simulink model "PTControl"  (Simulink 9.2)
settings: Solver=ode45  StartTime=0.0  StopTime=inf  RelTol=1e-3  EnableMultiTasking=on
libraries: CarMaker4SL x2
(part 2 of 3)

== system PTControl/CarMaker/IPG Vehicle/CarAndTrailer/Forces/Vehicle Forces ==
  Sync_In : Inport
  Bus Creator1 : BusCreator  Inputs=12
  Bus Creator8 : BusCreator  Inputs=16
  BusCreator1 : BusCreator  Inputs=4
  BusCreator2 : BusCreator  Inputs=9
  Demux : Demux  Outputs=16
  Demux1 : Demux  Outputs=12
  Demux2 : Demux  Outputs=13
  Forces : S-Function  FunctionName=CM_Sfun  Parameters='Forces'  SFunctionDeploymentMode=off  EnableBusSupport=off
  Terminator : Terminator
  Sync_Out : Outport
  Car.Virtual : Outport  Port=2
  Car.Aero : Outport  Port=3
  Car.Load : Outport  Port=4
  wires:
  BusCreator1/1 -> Terminator/1  "Aero IF (in)"
  Demux2/13 -> BusCreator2/9  "car Aero Trq_1 z"
  Demux2/12 -> BusCreator2/8  "car Aero Trq_1 y"
  Demux2/11 -> BusCreator2/7  "car Aero Trq_1 x"
  Demux2/10 -> BusCreator2/6  "car Aero Frc_1 z"
  Demux2/9 -> BusCreator2/5  "car Aero Frc_1 y"
  Demux2/8 -> BusCreator2/4  "car Aero Frc_1 x"
  Demux2/7 -> BusCreator2/3  "car Aero PoA_1 z"
  Demux2/6 -> BusCreator2/2  "car Aero PoA_1 y"
  Demux2/5 -> BusCreator2/1  "car Aero PoA_1 x"
  Demux2/4 -> BusCreator1/4  "car Aero tau_1"
  Demux2/3 -> BusCreator1/3  "car Aero ApproachVel_1 z"
  Demux2/2 -> BusCreator1/2  "car Aero ApproachVel_1 y"
  Demux2/1 -> BusCreator1/1  "car Aero ApproachVel_1 x"
  Demux/16 -> Bus Creator8/16  "Car Load_3 tz"
  Demux/15 -> Bus Creator8/15  "Car Load_3 ty"
  Demux/14 -> Bus Creator8/14  "Car Load_3 tx"
  Demux/13 -> Bus Creator8/13  "Car Load_3 mass"
  Demux1/12 -> Bus Creator1/12  "Car Virtual Trq_0 z"
  Demux1/11 -> Bus Creator1/11  "Car Virtual Trq_0 y"
  Demux1/10 -> Bus Creator1/10  "Car Virtual Trq_0 x"
  Demux1/9 -> Bus Creator1/9  "Car Virtual Trq_1 z"
  Demux1/8 -> Bus Creator1/8  "Car Virtual Trq_1 y"
  Demux1/7 -> Bus Creator1/7  "Car Virtual Trq_1 x"
  Demux1/6 -> Bus Creator1/6  "Car Virtual Frc_0 z"
  Demux1/5 -> Bus Creator1/5  "Car Virtual Frc_0 y"
  Demux1/4 -> Bus Creator1/4  "Car Virtual Frc_0 x"
  Sync_In/1 -> Forces/1
  Forces/1 -> Sync_Out/1
  BusCreator2/1 -> Car.Aero/1
  Demux1/1 -> Bus Creator1/1  "Car Virtual Frc_1 x"
  Demux1/2 -> Bus Creator1/2  "Car Virtual Frc_1 y"
  Demux1/3 -> Bus Creator1/3  "Car Virtual Frc_1 z"
  Forces/3 -> Demux2/1
  Forces/2 -> Demux1/1
  Bus Creator1/1 -> Car.Virtual/1
  Bus Creator8/1 -> Car.Load/1
  Demux/1 -> Bus Creator8/1  "Car Load_0 mass"
  Demux/2 -> Bus Creator8/2  "Car Load_0 tx"
  Demux/3 -> Bus Creator8/3  "Car Load_0 ty"
  Demux/4 -> Bus Creator8/4  "Car Load_0 tz"
  Demux/5 -> Bus Creator8/5  "Car Load_1 mass"
  Demux/6 -> Bus Creator8/6  "Car Load_1 tx"
  Demux/7 -> Bus Creator8/7  "Car Load_1 ty"
  Demux/8 -> Bus Creator8/8  "Car Load_1 tz"
  Demux/9 -> Bus Creator8/9  "Car Load_2 mass"
  Demux/10 -> Bus Creator8/10  "Car Load_2 tx"
  Demux/11 -> Bus Creator8/11  "Car Load_2 ty"
  Demux/12 -> Bus Creator8/12  "Car Load_2 tz"
  Forces/4 -> Demux/1

== system PTControl/CarMaker/IPG Vehicle/CarAndTrailer/Trailer/CreateBus Car.Hitch.FrcTrq ==
  In1 : Inport
  Bus Creator7 : BusCreator  Inputs=6
  Demux7 : Demux  Outputs=6
  Out1 : Outport
  wires:
  In1/1 -> Demux7/1
  Bus Creator7/1 -> Out1/1
  Demux7/6 -> Bus Creator7/6  "Car Hitch Trq2Car z"
  Demux7/5 -> Bus Creator7/5  "Car Hitch Trq2Car y"
  Demux7/4 -> Bus Creator7/4  "Car Hitch Trq2Car x"
  Demux7/3 -> Bus Creator7/3  "Car Hitch Frc2Car z"
  Demux7/2 -> Bus Creator7/2  "Car Hitch Frc2Car y"
  Demux7/1 -> Bus Creator7/1  "Car Hitch Frc2Car x"

== system PTControl/CarMaker/IPG Vehicle/CarAndTrailer/Trailer/CreateBus Vhcl.Motion ==
  In1 : Inport
  BusCreator : BusCreator  Inputs=15
  Demux : Demux  Outputs=15
  Out1 : Outport
  wires:
  Demux/15 -> BusCreator/15  "Vhcl YawAcc"
  Demux/14 -> BusCreator/14  "Vhcl YawVel"
  Demux/13 -> BusCreator/13  "Vhcl Yaw"
  Demux/12 -> BusCreator/12  "Vhcl PitchAcc"
  Demux/11 -> BusCreator/11  "Vhcl PitchVel"
  Demux/10 -> BusCreator/10  "Vhcl Pitch"
  Demux/9 -> BusCreator/9  "Vhcl RollAcc"
  Demux/8 -> BusCreator/8  "Vhcl RollVel"
  Demux/7 -> BusCreator/7  "Vhcl Roll"
  Demux/6 -> BusCreator/6  "Vhcl Hitch_Pos z"
  Demux/5 -> BusCreator/5  "Vhcl Hitch_Pos y"
  Demux/4 -> BusCreator/4  "Vhcl Hitch_Pos x"
  Demux/3 -> BusCreator/3  "Vhcl sRoad"
  Demux/2 -> BusCreator/2  "Vhcl Distance"
  Demux/1 -> BusCreator/1  "Vhcl v"
  In1/1 -> Demux/1
  BusCreator/1 -> Out1/1

== system PTControl/CarMaker/IPG Vehicle/CarAndTrailer/Trailer/CreateBus Vhcl.PoI ==
  In1 : Inport
  Bus Creator3 : BusCreator  Inputs=18
  Demux3 : Demux  Outputs=18
  Out1 : Outport
  wires:
  Demux3/18 -> Bus Creator3/18  "Vhcl PoI_GCS Elev"
  Demux3/17 -> Bus Creator3/17  "Vhcl PoI_GCS Lat"
  Demux3/16 -> Bus Creator3/16  "Vhcl PoI_GCS Long"
  Demux3/15 -> Bus Creator3/15  "Vhcl PoI_Acc_1 z"
  Demux3/14 -> Bus Creator3/14  "Vhcl PoI_Acc_1 y"
  Demux3/13 -> Bus Creator3/13  "Vhcl PoI_Acc_1 x"
  Demux3/12 -> Bus Creator3/12  "Vhcl PoI_Vel_1 z"
  Demux3/11 -> Bus Creator3/11  "Vhcl PoI_Vel_1 y"
  Demux3/10 -> Bus Creator3/10  "Vhcl PoI_Vel_1 x"
  Demux3/9 -> Bus Creator3/9  "Vhcl PoI_Acc z"
  Demux3/8 -> Bus Creator3/8  "Vhcl PoI_Acc y"
  Demux3/7 -> Bus Creator3/7  "Vhcl PoI_Acc x"
  Demux3/6 -> Bus Creator3/6  "Vhcl PoI_Vel z"
  Demux3/5 -> Bus Creator3/5  "Vhcl PoI_Vel y"
  Demux3/4 -> Bus Creator3/4  "Vhcl PoI_Vel x"
  Demux3/3 -> Bus Creator3/3  "Vhcl PoI_Pos z"
  Demux3/2 -> Bus Creator3/2  "Vhcl PoI_Pos y"
  In1/1 -> Demux3/1
  Bus Creator3/1 -> Out1/1
  Demux3/1 -> Bus Creator3/1  "Vhcl PoI_Pos x"

== system PTControl/CarMaker/IPG Vehicle/CarAndTrailer/Trailer/CreateBus Vhcl.Steering ==
  In1 : Inport
  Bus Creator3 : BusCreator  Inputs=4
  Demux : Demux
  Out1 : Outport
  wires:
  Bus Creator3/1 -> Out1/1
  Demux/1 -> Bus Creator3/1  "Vhcl Steering Ang"
  Demux/3 -> Bus Creator3/3  "Vhcl Steering AngAcc"
  Demux/2 -> Bus Creator3/2  "Vhcl Steering AngVel"
  Demux/4 -> Bus Creator3/4  "Vhcl Steering Trq"
  In1/1 -> Demux/1

== system PTControl/CarMaker/IPG Vehicle/CarAndTrailer/Trailer/CreateBus Vhcl.Wheel.FL ==
  In1 : Inport
  Bus Creator3 : BusCreator  Inputs=14
  Demux3 : Demux  Outputs=14
  Out1 : Outport
  wires:
  Demux3/14 -> Bus Creator3/14  "Vhcl Wheel FL Trq_WhlBearing"
  Demux3/13 -> Bus Creator3/13  "Vhcl Wheel FL Trq_T2W"
  Demux3/12 -> Bus Creator3/12  "Vhcl Wheel FL SideSlip"
  Demux3/11 -> Bus Creator3/11  "Vhcl Wheel FL LongSlip"
  Demux3/10 -> Bus Creator3/10  "Vhcl Wheel FL vBelt"
  Demux3/9 -> Bus Creator3/9  "Vhcl Wheel FL Fz"
  Demux3/8 -> Bus Creator3/8  "Vhcl Wheel FL Fy"
  Demux3/7 -> Bus Creator3/7  "Vhcl Wheel FL Fx"
  Demux3/6 -> Bus Creator3/6  "Vhcl Wheel FL r_zxy z"
  Demux3/5 -> Bus Creator3/5  "Vhcl Wheel FL r_zxy y"
  Demux3/4 -> Bus Creator3/4  "Vhcl Wheel FL r_zxy x"
  Demux3/3 -> Bus Creator3/3  "Vhcl Wheel FL t z"
  Demux3/2 -> Bus Creator3/2  "Vhcl Wheel FL t y"
  In1/1 -> Demux3/1
  Bus Creator3/1 -> Out1/1
  Demux3/1 -> Bus Creator3/1  "Vhcl Wheel FL t x"

== system PTControl/CarMaker/IPG Vehicle/CarAndTrailer/Trailer/CreateBus Vhcl.Wheel.FR ==
  In1 : Inport
  Bus Creator3 : BusCreator  Inputs=14
  Demux3 : Demux  Outputs=14
  Out1 : Outport
  wires:
  Demux3/14 -> Bus Creator3/14  "Vhcl Wheel FR Trq_WhlBearing"
  Demux3/13 -> Bus Creator3/13  "Vhcl Wheel FR Trq_T2W"
  Demux3/12 -> Bus Creator3/12  "Vhcl Wheel FR SideSlip"
  Demux3/11 -> Bus Creator3/11  "Vhcl Wheel FR LongSlip"
  Demux3/10 -> Bus Creator3/10  "Vhcl Wheel FR vBelt"
  Demux3/9 -> Bus Creator3/9  "Vhcl Wheel FR Fz"
  Demux3/8 -> Bus Creator3/8  "Vhcl Wheel FR Fy"
  Demux3/7 -> Bus Creator3/7  "Vhcl Wheel FR Fx"
  Demux3/6 -> Bus Creator3/6  "Vhcl Wheel FR r_zxy z"
  Demux3/5 -> Bus Creator3/5  "Vhcl Wheel FR r_zxy y"
  Demux3/4 -> Bus Creator3/4  "Vhcl Wheel FR r_zxy x"
  Demux3/3 -> Bus Creator3/3  "Vhcl Wheel FR t z"
  Demux3/2 -> Bus Creator3/2  "Vhcl Wheel FR t y"
  In1/1 -> Demux3/1
  Bus Creator3/1 -> Out1/1
  Demux3/1 -> Bus Creator3/1  "Vhcl Wheel FR t x"

== system PTControl/CarMaker/IPG Vehicle/CarAndTrailer/Trailer/CreateBus Vhcl.Wheel.RL ==
  In1 : Inport
  Bus Creator3 : BusCreator  Inputs=14
  Demux3 : Demux  Outputs=14
  Out1 : Outport
  wires:
  Demux3/14 -> Bus Creator3/14  "Vhcl Wheel RL Trq_WhlBearing"
  Demux3/13 -> Bus Creator3/13  "Vhcl Wheel RL Trq_T2W"
  Demux3/12 -> Bus Creator3/12  "Vhcl Wheel RL SideSlip"
  Demux3/11 -> Bus Creator3/11  "Vhcl Wheel RL LongSlip"
  Demux3/10 -> Bus Creator3/10  "Vhcl Wheel RL vBelt"
  Demux3/9 -> Bus Creator3/9  "Vhcl Wheel RL Fz"
  Demux3/8 -> Bus Creator3/8  "Vhcl Wheel RL Fy"
  Demux3/7 -> Bus Creator3/7  "Vhcl Wheel RL Fx"
  Demux3/6 -> Bus Creator3/6  "Vhcl Wheel RL r_zxy z"
  Demux3/5 -> Bus Creator3/5  "Vhcl Wheel RL r_zxy y"
  Demux3/4 -> Bus Creator3/4  "Vhcl Wheel RL r_zxy x"
  Demux3/3 -> Bus Creator3/3  "Vhcl Wheel RL t z"
  Demux3/2 -> Bus Creator3/2  "Vhcl Wheel RL t y"
  In1/1 -> Demux3/1
  Bus Creator3/1 -> Out1/1
  Demux3/1 -> Bus Creator3/1  "Vhcl Wheel RL t x"

== system PTControl/CarMaker/IPG Vehicle/CarAndTrailer/Trailer/CreateBus Vhcl.Wheel.RR ==
  In1 : Inport
  Bus Creator3 : BusCreator  Inputs=14
  Demux3 : Demux  Outputs=14
  Out1 : Outport
  wires:
  Demux3/14 -> Bus Creator3/14  "Vhcl Wheel RR Trq_WhlBearing"
  Demux3/13 -> Bus Creator3/13  "Vhcl Wheel RR Trq_T2W"
  Demux3/12 -> Bus Creator3/12  "Vhcl Wheel RR SideSlip"
  Demux3/11 -> Bus Creator3/11  "Vhcl Wheel RR LongSlip"
  Demux3/10 -> Bus Creator3/10  "Vhcl Wheel RR vBelt"
  Demux3/9 -> Bus Creator3/9  "Vhcl Wheel RR Fz"
  Demux3/8 -> Bus Creator3/8  "Vhcl Wheel RR Fy"
  Demux3/7 -> Bus Creator3/7  "Vhcl Wheel RR Fx"
  Demux3/6 -> Bus Creator3/6  "Vhcl Wheel RR r_zxy z"
  Demux3/5 -> Bus Creator3/5  "Vhcl Wheel RR r_zxy y"
  Demux3/4 -> Bus Creator3/4  "Vhcl Wheel RR r_zxy x"
  Demux3/3 -> Bus Creator3/3  "Vhcl Wheel RR t z"
  Demux3/2 -> Bus Creator3/2  "Vhcl Wheel RR t y"
  In1/1 -> Demux3/1
  Bus Creator3/1 -> Out1/1
  Demux3/1 -> Bus Creator3/1  "Vhcl Wheel RR t x"

== system PTControl/CarMaker/IPG Vehicle/PowerTrain/PTControl Example/CreateBus PTC ClutchOut ==
  In : Inport
  BusCreator : BusCreator  Inputs=3
  Demux : Demux  Outputs=3
  Out : Outport
  wires:
  Demux/3 -> BusCreator/3  "PTC ClutchOut Trq_out_trg"
  Demux/2 -> BusCreator/2  "PTC ClutchOut rotv_out_trg"
  Demux/1 -> BusCreator/1  "PTC ClutchOut Pos"
  BusCreator/1 -> Out/1
  In/1 -> Demux/1

== system PTControl/CarMaker/IPG Vehicle/PowerTrain/PTControl Example/CreateBus PTC EngineOut ==
  In : Inport
  BusCreator : BusCreator  Inputs=5
  Demux : Demux  Outputs=5
  Out : Outport
  wires:
  Demux/5 -> BusCreator/5  "PTC EngineOut rotv_trg"
  Demux/4 -> BusCreator/4  "PTC EngineOut Trq_trg"
  Demux/3 -> BusCreator/3  "PTC EngineOut Load"
  Demux/2 -> BusCreator/2  "PTC EngineOut FuelCutOff"
  Demux/1 -> BusCreator/1  "PTC EngineOut set_ISC"
  BusCreator/1 -> Out/1
  In/1 -> Demux/1

== system PTControl/CarMaker/IPG Vehicle/PowerTrain/PTControl Example/CreateBus PTC GearBoxM_Out0 ==
  In : Inport
  BusCreator : BusCreator  Inputs=12
  Demux : Demux  Outputs=12
  Out : Outport
  wires:
  Demux/12 -> BusCreator/12  "PTC GearBoxM_Out0 Clutch_dis Trq_out_trg"
  Demux/11 -> BusCreator/11  "PTC GearBoxM_Out0 Clutch_dis rotv_out_trg"
  Demux/10 -> BusCreator/10  "PTC GearBoxM_Out0 Clutch_dis Pos"
  Demux/9 -> BusCreator/9  "PTC GearBoxM_Out0 Clutch Trq_out_trg"
  Demux/8 -> BusCreator/8  "PTC GearBoxM_Out0 Clutch rotv_out_trg"
  Demux/7 -> BusCreator/7  "PTC GearBoxM_Out0 Clutch Pos"
  Demux/6 -> BusCreator/6  "PTC GearBoxM_Out0 Trq_out_trg"
  Demux/5 -> BusCreator/5  "PTC GearBoxM_Out0 rotv_in_trg"
  Demux/4 -> BusCreator/4  "PTC GearBoxM_Out0 i_trg"
  Demux/3 -> BusCreator/3  "PTC GearBoxM_Out0 set_ParkBrake"
  Demux/2 -> BusCreator/2  "PTC GearBoxM_Out0 GearNoTrg_dis"
  Demux/1 -> BusCreator/1  "PTC GearBoxM_Out0 GearNoTrg"
  BusCreator/1 -> Out/1
  In/1 -> Demux/1

== system PTControl/CarMaker/IPG Vehicle/PowerTrain/PTControl Example/CreateBus PTC GearBoxM_Out1 ==
  In : Inport
  BusCreator : BusCreator  Inputs=12
  Demux : Demux  Outputs=12
  Out : Outport
  wires:
  Demux/12 -> BusCreator/12  "PTC GearBoxM_Out1 Clutch_dis Trq_out_trg"
  Demux/11 -> BusCreator/11  "PTC GearBoxM_Out1 Clutch_dis rotv_out_trg"
  Demux/10 -> BusCreator/10  "PTC GearBoxM_Out1 Clutch_dis Pos"
  Demux/9 -> BusCreator/9  "PTC GearBoxM_Out1 Clutch Trq_out_trg"
  Demux/8 -> BusCreator/8  "PTC GearBoxM_Out1 Clutch rotv_out_trg"
  Demux/7 -> BusCreator/7  "PTC GearBoxM_Out1 Clutch Pos"
  Demux/6 -> BusCreator/6  "PTC GearBoxM_Out1 Trq_out_trg"
  Demux/5 -> BusCreator/5  "PTC GearBoxM_Out1 rotv_in_trg"
  Demux/4 -> BusCreator/4  "PTC GearBoxM_Out1 i_trg"
  Demux/3 -> BusCreator/3  "PTC GearBoxM_Out1 set_ParkBrake"
  Demux/2 -> BusCreator/2  "PTC GearBoxM_Out1 GearNoTrg_dis"
  Demux/1 -> BusCreator/1  "PTC GearBoxM_Out1 GearNoTrg"
  BusCreator/1 -> Out/1
  In/1 -> Demux/1

== system PTControl/CarMaker/IPG Vehicle/PowerTrain/PTControl Example/CreateBus PTC GearBoxM_Out2 ==
  In : Inport
  BusCreator : BusCreator  Inputs=12
  Demux : Demux  Outputs=12
  Out : Outport
  wires:
  Demux/12 -> BusCreator/12  "PTC GearBoxM_Out2 Clutch_dis Trq_out_trg"
  Demux/11 -> BusCreator/11  "PTC GearBoxM_Out2 Clutch_dis rotv_out_trg"
  Demux/10 -> BusCreator/10  "PTC GearBoxM_Out2 Clutch_dis Pos"
  Demux/9 -> BusCreator/9  "PTC GearBoxM_Out2 Clutch Trq_out_trg"
  Demux/8 -> BusCreator/8  "PTC GearBoxM_Out2 Clutch rotv_out_trg"
  Demux/7 -> BusCreator/7  "PTC GearBoxM_Out2 Clutch Pos"
  Demux/6 -> BusCreator/6  "PTC GearBoxM_Out2 Trq_out_trg"
  Demux/5 -> BusCreator/5  "PTC GearBoxM_Out2 rotv_in_trg"
  Demux/4 -> BusCreator/4  "PTC GearBoxM_Out2 i_trg"
  Demux/3 -> BusCreator/3  "PTC GearBoxM_Out2 set_ParkBrake"
  Demux/2 -> BusCreator/2  "PTC GearBoxM_Out2 GearNoTrg_dis"
  Demux/1 -> BusCreator/1  "PTC GearBoxM_Out2 GearNoTrg"
  BusCreator/1 -> Out/1
  In/1 -> Demux/1

== system PTControl/CarMaker/IPG Vehicle/PowerTrain/PTControl Example/CreateBus PTC GearBoxM_Out3 ==
  In : Inport
  BusCreator : BusCreator  Inputs=12
  Demux : Demux  Outputs=12
  Out : Outport
  wires:
  Demux/12 -> BusCreator/12  "PTC GearBoxM_Out3 Clutch_dis Trq_out_trg"
  Demux/11 -> BusCreator/11  "PTC GearBoxM_Out3 Clutch_dis rotv_out_trg"
  Demux/10 -> BusCreator/10  "PTC GearBoxM_Out3 Clutch_dis Pos"
  Demux/9 -> BusCreator/9  "PTC GearBoxM_Out3 Clutch Trq_out_trg"
  Demux/8 -> BusCreator/8  "PTC GearBoxM_Out3 Clutch rotv_out_trg"
  Demux/7 -> BusCreator/7  "PTC GearBoxM_Out3 Clutch Pos"
  Demux/6 -> BusCreator/6  "PTC GearBoxM_Out3 Trq_out_trg"
  Demux/5 -> BusCreator/5  "PTC GearBoxM_Out3 rotv_in_trg"
  Demux/4 -> BusCreator/4  "PTC GearBoxM_Out3 i_trg"
  Demux/3 -> BusCreator/3  "PTC GearBoxM_Out3 set_ParkBrake"
  Demux/2 -> BusCreator/2  "PTC GearBoxM_Out3 GearNoTrg_dis"
  Demux/1 -> BusCreator/1  "PTC GearBoxM_Out3 GearNoTrg"
  BusCreator/1 -> Out/1
  In/1 -> Demux/1

== system PTControl/CarMaker/IPG Vehicle/PowerTrain/PTControl Example/CreateBus PTC GearBoxOut ==
  In : Inport
  BusCreator : BusCreator  Inputs=12
  Demux : Demux  Outputs=12
  Out : Outport
  wires:
  Demux/12 -> BusCreator/12  "PTC GearBoxOut Clutch_dis Trq_out_trg"
  Demux/11 -> BusCreator/11  "PTC GearBoxOut Clutch_dis rotv_out_trg"
  Demux/10 -> BusCreator/10  "PTC GearBoxOut Clutch_dis Pos"
  Demux/9 -> BusCreator/9  "PTC GearBoxOut Clutch Trq_out_trg"
  Demux/8 -> BusCreator/8  "PTC GearBoxOut Clutch rotv_out_trg"
  Demux/7 -> BusCreator/7  "PTC GearBoxOut Clutch Pos"
  Demux/6 -> BusCreator/6  "PTC GearBoxOut Trq_out_trg"
  Demux/5 -> BusCreator/5  "PTC GearBoxOut rotv_in_trg"
  Demux/4 -> BusCreator/4  "PTC GearBoxOut i_trg"
  Demux/3 -> BusCreator/3  "PTC GearBoxOut set_ParkBrake"
  Demux/2 -> BusCreator/2  "PTC GearBoxOut GearNoTrg_dis"
  Demux/1 -> BusCreator/1  "PTC GearBoxOut GearNoTrg"
  BusCreator/1 -> Out/1
  In/1 -> Demux/1

== system PTControl/CarMaker/IPG Vehicle/PowerTrain/PTControl Example/CreateBus PTC ISGOut ==
  In : Inport
  BusCreator : BusCreator  Inputs=3
  Demux : Demux  Outputs=3
  Out : Outport
  wires:
  Demux/3 -> BusCreator/3  "PTC ISGOut rotv_trg"
  Demux/2 -> BusCreator/2  "PTC ISGOut Trq_trg"
  Demux/1 -> BusCreator/1  "PTC ISGOut Load"
  BusCreator/1 -> Out/1
  In/1 -> Demux/1

== system PTControl/CarMaker/IPG Vehicle/PowerTrain/PTControl Example/CreateBus PTC MiscOut ==
  In : Inport
  BusCreator : BusCreator  Inputs=4
  Demux : Demux
  Out : Outport
  wires:
  Demux/4 -> BusCreator/4  "PTC_Out Ignition"
  Demux/3 -> BusCreator/3  "PTC_Out StrategyMode"
  Demux/2 -> BusCreator/2  "PTC_Out OperationError"
  Demux/1 -> BusCreator/1  "PTC_Out OperationState"
  BusCreator/1 -> Out/1
  In/1 -> Demux/1

== system PTControl/CarMaker/IPG Vehicle/PowerTrain/PTControl Example/CreateBus PTC MotorOut0 ==
  In : Inport
  BusCreator : BusCreator  Inputs=3
  Demux : Demux  Outputs=3
  Gain : Gain  Gain=3
  Out : Outport
  wires:
  Demux/3 -> BusCreator/3  "PTC MotorOut0 rotv_trg"
  Demux/1 -> BusCreator/1  "PTC MotorOut0 Load"
  BusCreator/1 -> Out/1
  In/1 -> Demux/1
  Demux/2 -> Gain/1  "PTC MotorOut0 Trq_trg"
  Gain/1 -> BusCreator/2

== system PTControl/CarMaker/IPG Vehicle/PowerTrain/PTControl Example/CreateBus PTC MotorOut1 ==
  In : Inport
  BusCreator : BusCreator  Inputs=3
  Demux : Demux  Outputs=3
  Out : Outport
  wires:
  Demux/3 -> BusCreator/3  "PTC MotorOut1 rotv_trg"
  Demux/2 -> BusCreator/2  "PTC MotorOut1 Trq_trg"
  Demux/1 -> BusCreator/1  "PTC MotorOut1 Load"
  BusCreator/1 -> Out/1
  In/1 -> Demux/1

== system PTControl/CarMaker/IPG Vehicle/PowerTrain/PTControl Example/CreateBus PTC MotorOut2 ==
  In : Inport
  BusCreator : BusCreator  Inputs=3
  Demux : Demux  Outputs=3
  Out : Outport
  wires:
  Demux/3 -> BusCreator/3  "PTC MotorOut2 rotv_trg"
  Demux/2 -> BusCreator/2  "PTC MotorOut2 Trq_trg"
  Demux/1 -> BusCreator/1  "PTC MotorOut2 Load"
  BusCreator/1 -> Out/1
  In/1 -> Demux/1

== system PTControl/CarMaker/IPG Vehicle/PowerTrain/PTControl Example/CreateBus PTC MotorOut3 ==
  In : Inport
  BusCreator : BusCreator  Inputs=3
  Demux : Demux  Outputs=3
  Out : Outport
  wires:
  Demux/3 -> BusCreator/3  "PTC MotorOut3 rotv_trg"
  Demux/2 -> BusCreator/2  "PTC MotorOut3 Trq_trg"
  Demux/1 -> BusCreator/1  "PTC MotorOut3 Load"
  BusCreator/1 -> Out/1
  In/1 -> Demux/1

== system PTControl/CarMaker/IPG Vehicle/PowerTrain/PTControl Example/CreateBus PTC PwrSupplyOut ==
  In : Inport
  BusCreator : BusCreator  Inputs=1
  Demux : Demux  Outputs=1
  Out : Outport
  wires:
  Demux/1 -> BusCreator/1  "PTC PwrSupplyOut Pwr_HV1toLV_trg"
  BusCreator/1 -> Out/1
  In/1 -> Demux/1

== system PTControl/CarMaker/IPG Vehicle/PowerTrain/PTControl Example/CreateBus PTC WheelOut ==
  In : Inport
  BusCreator : BusCreator  Inputs=8
  Demux : Demux  Outputs=8
  Out : Outport
  wires:
  Demux/8 -> BusCreator/8  "PTC WheelOut_RR Trq_BrakeReg_max"
  Demux/7 -> BusCreator/7  "PTC WheelOut_RR Trq_BrakeReg"
  Demux/6 -> BusCreator/6  "PTC WheelOut_RL Trq_BrakeReg_max"
  Demux/5 -> BusCreator/5  "PTC WheelOut_RL Trq_BrakeReg"
  Demux/4 -> BusCreator/4  "PTC WheelOut_FR Trq_BrakeReg_max"
  Demux/3 -> BusCreator/3  "PTC WheelOut_FR Trq_BrakeReg"
  Demux/2 -> BusCreator/2  "PTC WheelOut_FL Trq_BrakeReg_max"
  Demux/1 -> BusCreator/1  "PTC WheelOut_FL Trq_BrakeReg"
  BusCreator/1 -> Out/1
  In/1 -> Demux/1

== system PTControl/CarMaker/IPG Vehicle/PowerTrain/PTControl Example/PTControl Example ==
  note: Minimalistic PTControl example model, that only works with
      | the 'Generic' powertrain and the 'Manual' gearbox.
  EngineIn : Inport
  VhclCtrl.PT : Inport  Port=2
  Bus Selector : BusSelector  OutputSignals=VhclCtrl Key,VhclCtrl Gas,VhclCtrl Clutch,VhclCtrl GearNo
  Bus Selector1 : BusSelector  OutputSignals=PTC EngineIn.PTC EngineIn Engine_on
  Define CM Dict : CarMaker4SL/Define CM Dict  xname=test  xmono=off  xtype=Double4  xdvaplace=None  xnstates=0  xfirststate=0  xinitial=0
  Engine : Subsystem
  ISG : Subsystem
  PTC : Subsystem
  Write CM Dict : CarMaker4SL/Write CM Dict  xname=test  xsync=off
  PTC MiscOut : Outport
  EngineOut : Outport  Port=2
  ISGOut : Outport  Port=3
  ClutchOut Pos : Outport  Port=4
  GearBoxOut GearNoTrg : Outport  Port=5
  wires:
  VhclCtrl.PT/1 -> Bus Selector/1
  EngineIn/1 -> Bus Selector1/1
  Engine/1(EngineOut) -> EngineOut/1
  Bus Selector1/1 -> Engine/2(Engine_on), PTC/2(Engine_on), Write CM Dict/1  "<PTC EngineIn Engine_on>"
  Bus Selector/2 -> Engine/1(Gas)  "<VhclCtrl Gas>"
  ISG/1(ISGOut) -> ISGOut/1
  PTC/1(PTC MiscOut) -> PTC MiscOut/1
  Bus Selector/4 -> GearBoxOut GearNoTrg/1  "<VhclCtrl GearNo>"
  Bus Selector/3 -> ClutchOut Pos/1  "<VhclCtrl Clutch>"
  Bus Selector/1 -> PTC/1(Key), ISG/1(Key)  "<VhclCtrl Key>"

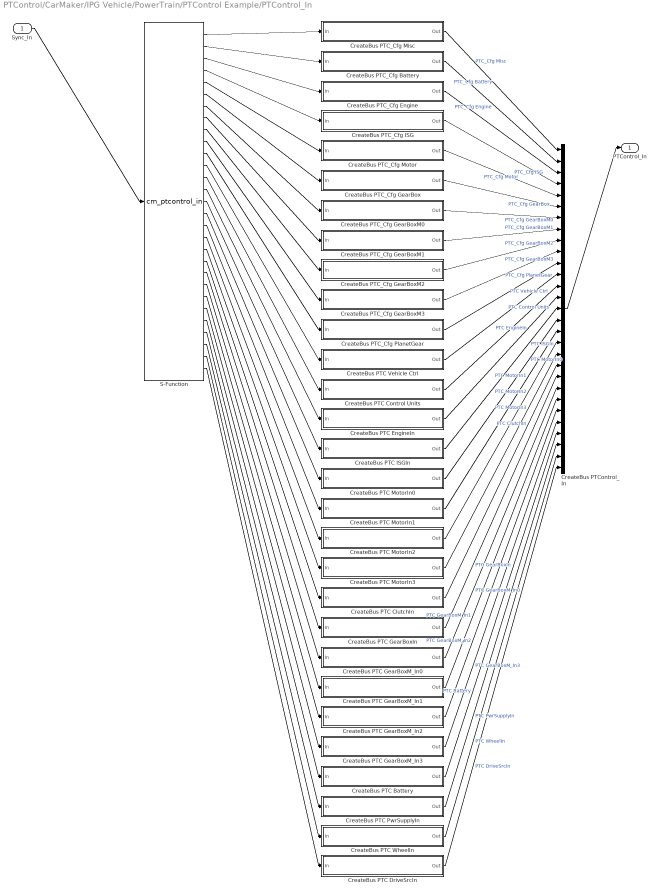
== system PTControl/CarMaker/IPG Vehicle/PowerTrain/PTControl Example/PTControl_In ==
  Sync_In : Inport
  CreateBus PTC Battery : Subsystem
  CreateBus PTC ClutchIn : Subsystem
  CreateBus PTC Control Units : Subsystem
  CreateBus PTC DriveSrcIn : Subsystem
  CreateBus PTC EngineIn : Subsystem
  CreateBus PTC GearBoxIn : Subsystem
  CreateBus PTC GearBoxM_In0 : Subsystem
  CreateBus PTC GearBoxM_In1 : Subsystem
  CreateBus PTC GearBoxM_In2 : Subsystem
  CreateBus PTC GearBoxM_In3 : Subsystem
  CreateBus PTC ISGIn : Subsystem
  CreateBus PTC MotorIn0 : Subsystem
  CreateBus PTC MotorIn1 : Subsystem
  CreateBus PTC MotorIn2 : Subsystem
  CreateBus PTC MotorIn3 : Subsystem
  CreateBus PTC PwrSupplyIn : Subsystem
  CreateBus PTC Vehicle Ctrl : Subsystem
  CreateBus PTC WheelIn : Subsystem
  CreateBus PTC_Cfg Battery : Subsystem
  CreateBus PTC_Cfg Engine : Subsystem
  CreateBus PTC_Cfg GearBox : Subsystem
  CreateBus PTC_Cfg GearBoxM0 : Subsystem
  CreateBus PTC_Cfg GearBoxM1 : Subsystem
  CreateBus PTC_Cfg GearBoxM2 : Subsystem
  CreateBus PTC_Cfg GearBoxM3 : Subsystem
  CreateBus PTC_Cfg ISG : Subsystem
  CreateBus PTC_Cfg Misc : Subsystem
  CreateBus PTC_Cfg Motor : Subsystem
  CreateBus PTC_Cfg PlanetGear : Subsystem
  CreateBus PTControl_In : BusCreator  Inputs=29
  S-Function : S-Function  FunctionName=cm_ptcontrol_in  SFunctionDeploymentMode=off  EnableBusSupport=off
  PTControl_In : Outport
  wires:
  CreateBus PTC DriveSrcIn/1(Out) -> CreateBus PTControl_In/29  "PTC DriveSrcIn"
  S-Function/29 -> CreateBus PTC DriveSrcIn/1(In)
  CreateBus PTC WheelIn/1(Out) -> CreateBus PTControl_In/28  "PTC WheelIn"
  S-Function/28 -> CreateBus PTC WheelIn/1(In)
  CreateBus PTC PwrSupplyIn/1(Out) -> CreateBus PTControl_In/27  "PTC PwrSupplyIn"
  S-Function/27 -> CreateBus PTC PwrSupplyIn/1(In)
  CreateBus PTC Battery/1(Out) -> CreateBus PTControl_In/26  "PTC Battery"
  S-Function/26 -> CreateBus PTC Battery/1(In)
  CreateBus PTC GearBoxM_In3/1(Out) -> CreateBus PTControl_In/25  "PTC GearBoxM_In3"
  S-Function/25 -> CreateBus PTC GearBoxM_In3/1(In)
  CreateBus PTC GearBoxM_In2/1(Out) -> CreateBus PTControl_In/24  "PTC GearBoxM_In2"
  S-Function/24 -> CreateBus PTC GearBoxM_In2/1(In)
  CreateBus PTC GearBoxM_In1/1(Out) -> CreateBus PTControl_In/23  "PTC GearBoxM_In1"
  S-Function/23 -> CreateBus PTC GearBoxM_In1/1(In)
  CreateBus PTC GearBoxM_In0/1(Out) -> CreateBus PTControl_In/22  "PTC GearBoxM_In0"
  S-Function/22 -> CreateBus PTC GearBoxM_In0/1(In)
  CreateBus PTC GearBoxIn/1(Out) -> CreateBus PTControl_In/21  "PTC GearBoxIn"
  S-Function/21 -> CreateBus PTC GearBoxIn/1(In)
  CreateBus PTC ClutchIn/1(Out) -> CreateBus PTControl_In/20  "PTC ClutchIn"
  S-Function/20 -> CreateBus PTC ClutchIn/1(In)
  CreateBus PTC MotorIn3/1(Out) -> CreateBus PTControl_In/19  "PTC MotorIn3"
  S-Function/19 -> CreateBus PTC MotorIn3/1(In)
  CreateBus PTC MotorIn2/1(Out) -> CreateBus PTControl_In/18  "PTC MotorIn2"
  S-Function/18 -> CreateBus PTC MotorIn2/1(In)
  CreateBus PTC MotorIn1/1(Out) -> CreateBus PTControl_In/17  "PTC MotorIn1"
  S-Function/17 -> CreateBus PTC MotorIn1/1(In)
  CreateBus PTC MotorIn0/1(Out) -> CreateBus PTControl_In/16  "PTC MotorIn0"
  S-Function/16 -> CreateBus PTC MotorIn0/1(In)
  CreateBus PTC ISGIn/1(Out) -> CreateBus PTControl_In/15  "PTC ISGIn"
  S-Function/15 -> CreateBus PTC ISGIn/1(In)
  CreateBus PTC EngineIn/1(Out) -> CreateBus PTControl_In/14  "PTC EngineIn"
  S-Function/14 -> CreateBus PTC EngineIn/1(In)
  CreateBus PTC Control Units/1(Out) -> CreateBus PTControl_In/13  "PTC Control Units"
  S-Function/13 -> CreateBus PTC Control Units/1(In)
  CreateBus PTC Vehicle Ctrl/1(Out) -> CreateBus PTControl_In/12  "PTC Vehicle Ctrl"
  S-Function/12 -> CreateBus PTC Vehicle Ctrl/1(In)
  CreateBus PTC_Cfg PlanetGear/1(Out) -> CreateBus PTControl_In/11  "PTC_Cfg PlanetGear"
  S-Function/11 -> CreateBus PTC_Cfg PlanetGear/1(In)
  CreateBus PTC_Cfg GearBoxM3/1(Out) -> CreateBus PTControl_In/10  "PTC_Cfg GearBoxM3"
  S-Function/10 -> CreateBus PTC_Cfg GearBoxM3/1(In)
  CreateBus PTC_Cfg GearBoxM2/1(Out) -> CreateBus PTControl_In/9  "PTC_Cfg GearBoxM2"
  S-Function/9 -> CreateBus PTC_Cfg GearBoxM2/1(In)
  CreateBus PTC_Cfg GearBoxM1/1(Out) -> CreateBus PTControl_In/8  "PTC_Cfg GearBoxM1"
  S-Function/8 -> CreateBus PTC_Cfg GearBoxM1/1(In)
  CreateBus PTC_Cfg GearBoxM0/1(Out) -> CreateBus PTControl_In/7  "PTC_Cfg GearBoxM0"
  S-Function/7 -> CreateBus PTC_Cfg GearBoxM0/1(In)
  CreateBus PTC_Cfg GearBox/1(Out) -> CreateBus PTControl_In/6  "PTC_Cfg GearBox"
  S-Function/6 -> CreateBus PTC_Cfg GearBox/1(In)
  CreateBus PTC_Cfg Motor/1(Out) -> CreateBus PTControl_In/5  "PTC_Cfg Motor"
  S-Function/5 -> CreateBus PTC_Cfg Motor/1(In)
  CreateBus PTC_Cfg ISG/1(Out) -> CreateBus PTControl_In/4  "PTC_Cfg ISG"
  S-Function/4 -> CreateBus PTC_Cfg ISG/1(In)
  CreateBus PTC_Cfg Engine/1(Out) -> CreateBus PTControl_In/3  "PTC_Cfg Engine"
  S-Function/3 -> CreateBus PTC_Cfg Engine/1(In)
  CreateBus PTC_Cfg Battery/1(Out) -> CreateBus PTControl_In/2  "PTC_Cfg Battery"
  S-Function/2 -> CreateBus PTC_Cfg Battery/1(In)
  CreateBus PTC_Cfg Misc/1(Out) -> CreateBus PTControl_In/1  "PTC_Cfg Misc"
  S-Function/1 -> CreateBus PTC_Cfg Misc/1(In)
  CreateBus PTControl_In/1 -> PTControl_In/1
  Sync_In/1 -> S-Function/1

== system PTControl/CarMaker/IPG Vehicle/PowerTrain/PTControl Example/PTControl_Out ==
  PTC MiscOut : Inport
  PTC EngineOut : Inport  Port=2
  PTC ISGOut : Inport  Port=3
  PTC MotorOut0 : Inport  Port=4
  PTC MotorOut1 : Inport  Port=5
  PTC MotorOut2 : Inport  Port=6
  PTC MotorOut3 : Inport  Port=7
  PTC ClutchOut : Inport  Port=8
  PTC GearBoxOut : Inport  Port=9
  PTC GearBoxM_Out0 : Inport  Port=10
  PTC GearBoxM_Out1 : Inport  Port=11
  PTC GearBoxM_Out2 : Inport  Port=12
  PTC GearBoxM_Out3 : Inport  Port=13
  PTC PwrSupplyOut : Inport  Port=14
  PTC WheelOut : Inport  Port=15
  PTControl_Out : S-Function  FunctionName=cm_ptcontrol_out  SFunctionDeploymentMode=off  EnableBusSupport=off
  wires:
  PTC WheelOut/1 -> PTControl_Out/15
  PTC PwrSupplyOut/1 -> PTControl_Out/14
  PTC GearBoxM_Out3/1 -> PTControl_Out/13
  PTC GearBoxM_Out2/1 -> PTControl_Out/12
  PTC GearBoxM_Out1/1 -> PTControl_Out/11
  PTC GearBoxM_Out0/1 -> PTControl_Out/10
  PTC GearBoxOut/1 -> PTControl_Out/9
  PTC ClutchOut/1 -> PTControl_Out/8
  PTC MotorOut3/1 -> PTControl_Out/7
  PTC MotorOut2/1 -> PTControl_Out/6
  PTC MotorOut1/1 -> PTControl_Out/5
  PTC MotorOut0/1 -> PTControl_Out/4
  PTC ISGOut/1 -> PTControl_Out/3
  PTC EngineOut/1 -> PTControl_Out/2
  PTC MiscOut/1 -> PTControl_Out/1

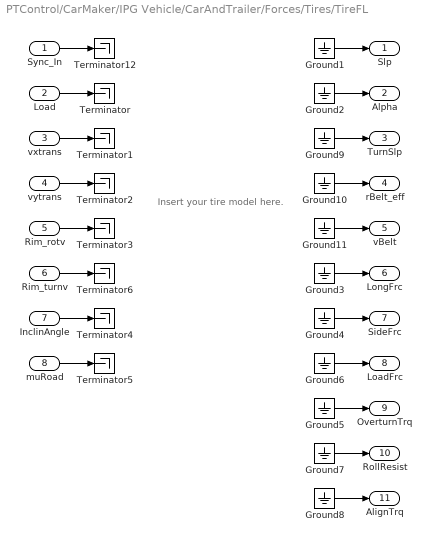
== system PTControl/CarMaker/IPG Vehicle/CarAndTrailer/Forces/Tires/TireFL ==
  note: Insert your tire model here.
  Sync_In : Inport
  Load : Inport  Port=2
  vxtrans : Inport  Port=3
  vytrans : Inport  Port=4
  Rim_rotv : Inport  Port=5
  Rim_turnv : Inport  Port=6
  InclinAngle : Inport  Port=7
  muRoad : Inport  Port=8
  Ground{1..11} (11 alike) : Ground
  Terminator{,1..6,12} (8 alike) : Terminator
  Slp : Outport
  Alpha : Outport  Port=2
  TurnSlp : Outport  Port=3
  rBelt_eff : Outport  Port=4
  vBelt : Outport  Port=5
  LongFrc : Outport  Port=6
  SideFrc : Outport  Port=7
  LoadFrc : Outport  Port=8
  OverturnTrq : Outport  Port=9
  RollResist : Outport  Port=10
  AlignTrq : Outport  Port=11
  wires:
  Ground11/1 -> vBelt/1
  Ground10/1 -> rBelt_eff/1
  Ground9/1 -> TurnSlp/1
  Rim_turnv/1 -> Terminator6/1
  Sync_In/1 -> Terminator12/1
  Ground2/1 -> Alpha/1
  Ground3/1 -> LongFrc/1
  Ground4/1 -> SideFrc/1
  Ground5/1 -> OverturnTrq/1
  vxtrans/1 -> Terminator1/1
  vytrans/1 -> Terminator2/1
  Rim_rotv/1 -> Terminator3/1
  InclinAngle/1 -> Terminator4/1
  muRoad/1 -> Terminator5/1
  Load/1 -> Terminator/1
  Ground1/1 -> Slp/1
  Ground6/1 -> LoadFrc/1
  Ground7/1 -> RollResist/1
  Ground8/1 -> AlignTrq/1

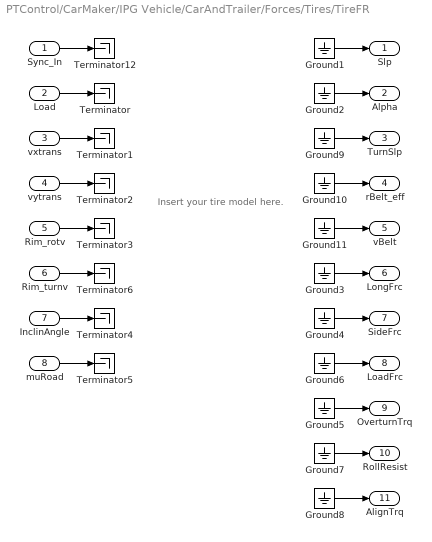
== system PTControl/CarMaker/IPG Vehicle/CarAndTrailer/Forces/Tires/TireFR ==
  note: Insert your tire model here.
  Sync_In : Inport
  Load : Inport  Port=2
  vxtrans : Inport  Port=3
  vytrans : Inport  Port=4
  Rim_rotv : Inport  Port=5
  Rim_turnv : Inport  Port=6
  InclinAngle : Inport  Port=7
  muRoad : Inport  Port=8
  Ground{1..11} (11 alike) : Ground
  Terminator{,1..6,12} (8 alike) : Terminator
  Slp : Outport
  Alpha : Outport  Port=2
  TurnSlp : Outport  Port=3
  rBelt_eff : Outport  Port=4
  vBelt : Outport  Port=5
  LongFrc : Outport  Port=6
  SideFrc : Outport  Port=7
  LoadFrc : Outport  Port=8
  OverturnTrq : Outport  Port=9
  RollResist : Outport  Port=10
  AlignTrq : Outport  Port=11
  wires:
  Ground11/1 -> vBelt/1
  Ground10/1 -> rBelt_eff/1
  Ground9/1 -> TurnSlp/1
  Rim_turnv/1 -> Terminator6/1
  Sync_In/1 -> Terminator12/1
  Ground2/1 -> Alpha/1
  Ground3/1 -> LongFrc/1
  Ground4/1 -> SideFrc/1
  Ground5/1 -> OverturnTrq/1
  vxtrans/1 -> Terminator1/1
  vytrans/1 -> Terminator2/1
  Rim_rotv/1 -> Terminator3/1
  InclinAngle/1 -> Terminator4/1
  muRoad/1 -> Terminator5/1
  Load/1 -> Terminator/1
  Ground1/1 -> Slp/1
  Ground6/1 -> LoadFrc/1
  Ground7/1 -> RollResist/1
  Ground8/1 -> AlignTrq/1

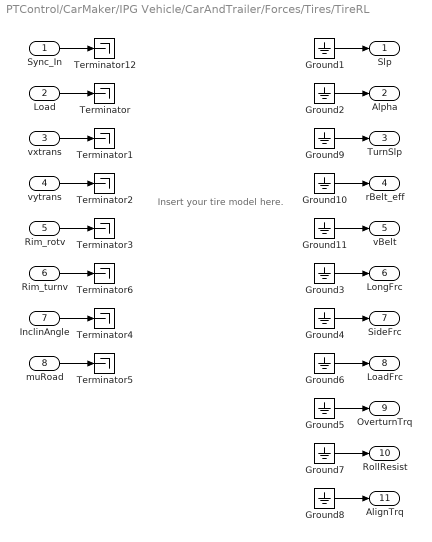
== system PTControl/CarMaker/IPG Vehicle/CarAndTrailer/Forces/Tires/TireRL ==
  note: Insert your tire model here.
  Sync_In : Inport
  Load : Inport  Port=2
  vxtrans : Inport  Port=3
  vytrans : Inport  Port=4
  Rim_rotv : Inport  Port=5
  Rim_turnv : Inport  Port=6
  InclinAngle : Inport  Port=7
  muRoad : Inport  Port=8
  Ground{1..11} (11 alike) : Ground
  Terminator{,1..6,12} (8 alike) : Terminator
  Slp : Outport
  Alpha : Outport  Port=2
  TurnSlp : Outport  Port=3
  rBelt_eff : Outport  Port=4
  vBelt : Outport  Port=5
  LongFrc : Outport  Port=6
  SideFrc : Outport  Port=7
  LoadFrc : Outport  Port=8
  OverturnTrq : Outport  Port=9
  RollResist : Outport  Port=10
  AlignTrq : Outport  Port=11
  wires:
  Ground11/1 -> vBelt/1
  Ground10/1 -> rBelt_eff/1
  Ground9/1 -> TurnSlp/1
  Rim_turnv/1 -> Terminator6/1
  Sync_In/1 -> Terminator12/1
  Ground2/1 -> Alpha/1
  Ground3/1 -> LongFrc/1
  Ground4/1 -> SideFrc/1
  Ground5/1 -> OverturnTrq/1
  vxtrans/1 -> Terminator1/1
  vytrans/1 -> Terminator2/1
  Rim_rotv/1 -> Terminator3/1
  InclinAngle/1 -> Terminator4/1
  muRoad/1 -> Terminator5/1
  Load/1 -> Terminator/1
  Ground1/1 -> Slp/1
  Ground6/1 -> LoadFrc/1
  Ground7/1 -> RollResist/1
  Ground8/1 -> AlignTrq/1

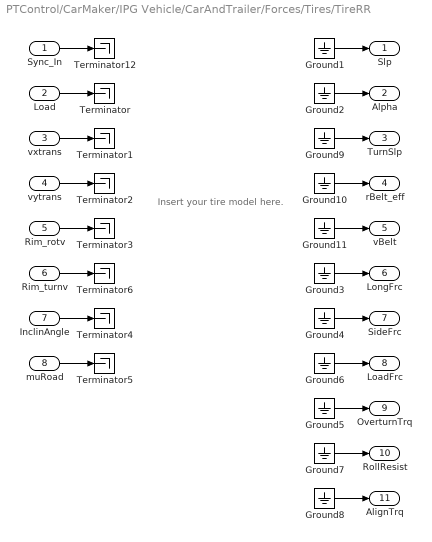
== system PTControl/CarMaker/IPG Vehicle/CarAndTrailer/Forces/Tires/TireRR ==
  note: Insert your tire model here.
  Sync_In : Inport
  Load : Inport  Port=2
  vxtrans : Inport  Port=3
  vytrans : Inport  Port=4
  Rim_rotv : Inport  Port=5
  Rim_turnv : Inport  Port=6
  InclinAngle : Inport  Port=7
  muRoad : Inport  Port=8
  Ground{1..11} (11 alike) : Ground
  Terminator{,1..6,12} (8 alike) : Terminator
  Slp : Outport
  Alpha : Outport  Port=2
  TurnSlp : Outport  Port=3
  rBelt_eff : Outport  Port=4
  vBelt : Outport  Port=5
  LongFrc : Outport  Port=6
  SideFrc : Outport  Port=7
  LoadFrc : Outport  Port=8
  OverturnTrq : Outport  Port=9
  RollResist : Outport  Port=10
  AlignTrq : Outport  Port=11
  wires:
  Ground11/1 -> vBelt/1
  Ground10/1 -> rBelt_eff/1
  Ground9/1 -> TurnSlp/1
  Rim_turnv/1 -> Terminator6/1
  Sync_In/1 -> Terminator12/1
  Ground2/1 -> Alpha/1
  Ground3/1 -> LongFrc/1
  Ground4/1 -> SideFrc/1
  Ground5/1 -> OverturnTrq/1
  vxtrans/1 -> Terminator1/1
  vytrans/1 -> Terminator2/1
  Rim_rotv/1 -> Terminator3/1
  InclinAngle/1 -> Terminator4/1
  muRoad/1 -> Terminator5/1
  Load/1 -> Terminator/1
  Ground1/1 -> Slp/1
  Ground6/1 -> LoadFrc/1
  Ground7/1 -> RollResist/1
  Ground8/1 -> AlignTrq/1

== system PTControl/CarMaker/IPG Vehicle/PowerTrain/PTControl Example/PTControl Example/Engine ==
  Gas : Inport
  Engine_on : Inport  Port=2
  Constant : Constant
  Constant1 : Constant  Value=0
  Constant3 : Constant  Value=0
  Mux : Mux  Inputs=5
  NOTSET0 : Constant  Value=-99999
  NOTSET1 : Constant  Value=-99999
  NOTSET2 : Constant  Value=-99999
  Switch : Switch  Criteria=u2 ~= 0
  Switch1 : Switch  Criteria=u2 ~= 0
  EngineOut : Outport
  wires:
  Constant/1 -> Switch/1
  Mux/1 -> EngineOut/1
  Constant1/1 -> Switch/3
  Engine_on/1 -> Switch/2, Switch1/2
  Gas/1 -> Switch1/1
  Constant3/1 -> Switch1/3
  NOTSET1/1 -> Mux/5  "rotv_trg"
  NOTSET2/1 -> Mux/4  "Trq_trg"
  Switch1/1 -> Mux/3  "Load"
  NOTSET0/1 -> Mux/2  "FuelCutOff"
  Switch/1 -> Mux/1  "set_ISC"

== system PTControl/CarMaker/IPG Vehicle/PowerTrain/PTControl Example/PTControl Example/ISG ==
  Key : Inport
  Constant : Constant
  Constant1 : Constant  Value=0
  KeyPos_KeyIn_Starter : Constant  Value=4
  Mux : Mux  Inputs=3
  NOTSET : Constant  Value=-99999
  NOTSET1 : Constant  Value=-99999
  Relational Operator1 : RelationalOperator  Operator===  OutDataTypeStr=boolean  RndMeth=Nearest
  Switch : Switch  Criteria=u2 ~= 0
  ISGOut : Outport
  wires:
  KeyPos_KeyIn_Starter/1 -> Relational Operator1/2
  Constant/1 -> Switch/1
  Constant1/1 -> Switch/3
  Relational Operator1/1 -> Switch/2
  Key/1 -> Relational Operator1/1
  Switch/1 -> Mux/1  "Load"
  NOTSET/1 -> Mux/2  "Trq_trg"
  NOTSET1/1 -> Mux/3  "rotv_trg"
  Mux/1 -> ISGOut/1

== system PTControl/CarMaker/IPG Vehicle/PowerTrain/PTControl Example/PTControl Example/PTC ==
  Key : Inport
  Engine_on : Inport  Port=2
  Constant : Constant
  Constant1 : Constant  Value=0
  Ground : Ground
  KeyPos2OperState : Lookup  InputValues=[0 1 2 3 4 5 6 7 8 9]  Table=[0 1 2 3 3 3 3 3 3 3]
  KeyPos_KeyIn_PowerOn : Constant  Value=3
  Logical Operator : Logic  AllPortsSameDT=off  OutDataTypeStr=boolean
  Mode_EngineDrive : Constant  Value=8
  Mux : Mux
  OperState_Driving : Constant  Value=4
  OperState_PowerOn : Constant  Value=3
  Relational Operator : RelationalOperator  OutDataTypeStr=boolean  RndMeth=Nearest
  Relational Operator1 : RelationalOperator  OutDataTypeStr=boolean  RndMeth=Nearest
  Switch : Switch  Criteria=u2 ~= 0
  Switch1 : Switch  Criteria=u2 ~= 0
  PTC MiscOut : Outport
  wires:
  KeyPos_KeyIn_PowerOn/1 -> Relational Operator/2
  Ground/1 -> Mux/2  "OperationError"
  Mux/1 -> PTC MiscOut/1
  Key/1 -> KeyPos2OperState/1, Relational Operator/1
  Constant/1 -> Switch/1
  Constant1/1 -> Switch/3
  Relational Operator/1 -> Switch/2  "Ignition"
  OperState_Driving/1 -> Switch1/1
  Switch1/1 -> Mux/1  "OperationState"
  KeyPos2OperState/1 -> Relational Operator1/1, Switch1/3  "OperationState"
  Logical Operator/1 -> Switch1/2
  Engine_on/1 -> Logical Operator/1
  Relational Operator1/1 -> Logical Operator/2
  OperState_PowerOn/1 -> Relational Operator1/2
  Switch/1 -> Mux/4  "Ignition"
  Mode_EngineDrive/1 -> Mux/3

== system PTControl/CarMaker/IPG Vehicle/PowerTrain/PTControl Example/PTControl_In/CreateBus PTC Battery ==
  In : Inport
  BusCreator : BusCreator  Inputs=14
  Demux : Demux  Outputs=14
  Out : Outport
  wires:
  Demux/14 -> BusCreator/14  "PTC BattHVIn Pwr_max"
  Demux/13 -> BusCreator/13  "PTC BattHVIn Energy"
  Demux/12 -> BusCreator/12  "PTC BattHVIn Temp"
  Demux/11 -> BusCreator/11  "PTC BattHVIn AOC"
  Demux/10 -> BusCreator/10  "PTC BattHVIn Current"
  Demux/9 -> BusCreator/9  "PTC BattHVIn SOH"
  Demux/8 -> BusCreator/8  "PTC BattHVIn SOC"
  Demux/7 -> BusCreator/7  "PTC BattLVIn Pwr_max"
  Demux/6 -> BusCreator/6  "PTC BattLVIn Energy"
  Demux/5 -> BusCreator/5  "PTC BattLVIn Temp"
  Demux/4 -> BusCreator/4  "PTC BattLVIn AOC"
  Demux/3 -> BusCreator/3  "PTC BattLVIn Current"
  Demux/2 -> BusCreator/2  "PTC BattLVIn SOH"
  Demux/1 -> BusCreator/1  "PTC BattLVIn SOC"
  BusCreator/1 -> Out/1
  In/1 -> Demux/1

== system PTControl/CarMaker/IPG Vehicle/PowerTrain/PTControl Example/PTControl_In/CreateBus PTC ClutchIn ==
  In : Inport
  BusCreator : BusCreator  Inputs=6
  Demux : Demux  Outputs=6
  Out : Outport
  wires:
  Demux/6 -> BusCreator/6  "PTC ClutchIn i_TrqIn2Out"
  Demux/5 -> BusCreator/5  "PTC ClutchIn Trq_out"
  Demux/4 -> BusCreator/4  "PTC ClutchIn Trq_in"
  Demux/3 -> BusCreator/3  "PTC ClutchIn rotv_out"
  Demux/2 -> BusCreator/2  "PTC ClutchIn rotv_in"
  Demux/1 -> BusCreator/1  "PTC ClutchIn Pos"
  BusCreator/1 -> Out/1
  In/1 -> Demux/1

== system PTControl/CarMaker/IPG Vehicle/PowerTrain/PTControl Example/PTControl_In/CreateBus PTC Control Units ==
  In : Inport
  BusCreator : BusCreator  Inputs=4
  Demux : Demux
  Out : Outport
  wires:
  Demux/4 -> BusCreator/4  "PTC BCU_Status"
  Demux/3 -> BusCreator/3  "PTC TCU_Status"
  Demux/2 -> BusCreator/2  "PTC MCU_Status"
  Demux/1 -> BusCreator/1  "PTC ECU_Status"
  BusCreator/1 -> Out/1
  In/1 -> Demux/1

== system PTControl/CarMaker/IPG Vehicle/PowerTrain/PTControl Example/PTControl_In/CreateBus PTC DriveSrcIn ==
  In : Inport
  BusCreator : BusCreator  Inputs=4
  Demux : Demux
  Out : Outport
  wires:
  Demux/4 -> BusCreator/4  "PTC DriveSrcIn_d3 Trq_DriveSrc_trg"
  Demux/3 -> BusCreator/3  "PTC DriveSrcIn_d2 Trq_DriveSrc_trg"
  Demux/2 -> BusCreator/2  "PTC DriveSrcIn_d1 Trq_DriveSrc_trg"
  Demux/1 -> BusCreator/1  "PTC DriveSrcIn_d0 Trq_DriveSrc_trg"
  BusCreator/1 -> Out/1
  In/1 -> Demux/1

== system PTControl/CarMaker/IPG Vehicle/PowerTrain/PTControl Example/PTControl_In/CreateBus PTC EngineIn ==
  In : Inport
  BusCreator : BusCreator  Inputs=7
  Demux : Demux  Outputs=7
  Out : Outport
  wires:
  Demux/7 -> BusCreator/7  "PTC EngineIn FuelFlow"
  Demux/6 -> BusCreator/6  "PTC EngineIn TrqOpt"
  Demux/5 -> BusCreator/5  "PTC EngineIn TrqFull"
  Demux/4 -> BusCreator/4  "PTC EngineIn TrqDrag"
  Demux/3 -> BusCreator/3  "PTC EngineIn Trq"
  Demux/2 -> BusCreator/2  "PTC EngineIn rotv"
  Demux/1 -> BusCreator/1  "PTC EngineIn Engine_on"
  BusCreator/1 -> Out/1
  In/1 -> Demux/1

== system PTControl/CarMaker/IPG Vehicle/PowerTrain/PTControl Example/PTControl_In/CreateBus PTC GearBoxIn ==
  In : Inport
  BusCreator : BusCreator  Inputs=20
  Demux : Demux  Outputs=20
  Out : Outport
  wires:
  Demux/20 -> BusCreator/20  "PTC GearBoxIn Clutch_dis i_TrqIn2Out"
  Demux/19 -> BusCreator/19  "PTC GearBoxIn Clutch_dis Trq_out"
  Demux/18 -> BusCreator/18  "PTC GearBoxIn Clutch_dis Trq_in"
  Demux/17 -> BusCreator/17  "PTC GearBoxIn Clutch_dis rotv_out"
  Demux/16 -> BusCreator/16  "PTC GearBoxIn Clutch_dis rotv_in"
  Demux/15 -> BusCreator/15  "PTC GearBoxIn Clutch_dis Pos"
  Demux/14 -> BusCreator/14  "PTC GearBoxIn Clutch i_TrqIn2Out"
  Demux/13 -> BusCreator/13  "PTC GearBoxIn Clutch Trq_out"
  Demux/12 -> BusCreator/12  "PTC GearBoxIn Clutch Trq_in"
  Demux/11 -> BusCreator/11  "PTC GearBoxIn Clutch rotv_out"
  Demux/10 -> BusCreator/10  "PTC GearBoxIn Clutch rotv_in"
  Demux/9 -> BusCreator/9  "PTC GearBoxIn Clutch Pos"
  Demux/8 -> BusCreator/8  "PTC GearBoxIn Trq_out"
  Demux/7 -> BusCreator/7  "PTC GearBoxIn Trq_in"
  Demux/6 -> BusCreator/6  "PTC GearBoxIn rotv_out"
  Demux/5 -> BusCreator/5  "PTC GearBoxIn rotv_in"
  Demux/4 -> BusCreator/4  "PTC GearBoxIn i"
  Demux/3 -> BusCreator/3  "PTC GearBoxIn Trq_DriveSrc_trg"
  Demux/2 -> BusCreator/2  "PTC GearBoxIn GearNo_dis"
  Demux/1 -> BusCreator/1  "PTC GearBoxIn GearNo"
  BusCreator/1 -> Out/1
  In/1 -> Demux/1

== system PTControl/CarMaker/IPG Vehicle/PowerTrain/PTControl Example/PTControl_In/CreateBus PTC GearBoxM_In0 ==
  In : Inport
  BusCreator : BusCreator  Inputs=20
  Demux : Demux  Outputs=20
  Out : Outport
  wires:
  Demux/20 -> BusCreator/20  "PTC GearBoxM_In0 Clutch_dis i_TrqIn2Out"
  Demux/19 -> BusCreator/19  "PTC GearBoxM_In0 Clutch_dis Trq_out"
  Demux/18 -> BusCreator/18  "PTC GearBoxM_In0 Clutch_dis Trq_in"
  Demux/17 -> BusCreator/17  "PTC GearBoxM_In0 Clutch_dis rotv_out"
  Demux/16 -> BusCreator/16  "PTC GearBoxM_In0 Clutch_dis rotv_in"
  Demux/15 -> BusCreator/15  "PTC GearBoxM_In0 Clutch_dis Pos"
  Demux/14 -> BusCreator/14  "PTC GearBoxM_In0 Clutch i_TrqIn2Out"
  Demux/13 -> BusCreator/13  "PTC GearBoxM_In0 Clutch Trq_out"
  Demux/12 -> BusCreator/12  "PTC GearBoxM_In0 Clutch Trq_in"
  Demux/11 -> BusCreator/11  "PTC GearBoxM_In0 Clutch rotv_out"
  Demux/10 -> BusCreator/10  "PTC GearBoxM_In0 Clutch rotv_in"
  Demux/9 -> BusCreator/9  "PTC GearBoxM_In0 Clutch Pos"
  Demux/8 -> BusCreator/8  "PTC GearBoxM_In0 Trq_out"
  Demux/7 -> BusCreator/7  "PTC GearBoxM_In0 Trq_in"
  Demux/6 -> BusCreator/6  "PTC GearBoxM_In0 rotv_out"
  Demux/5 -> BusCreator/5  "PTC GearBoxM_In0 rotv_in"
  Demux/4 -> BusCreator/4  "PTC GearBoxM_In0 i"
  Demux/3 -> BusCreator/3  "PTC GearBoxM_In0 Trq_DriveSrc_trg"
  Demux/2 -> BusCreator/2  "PTC GearBoxM_In0 GearNo_dis"
  Demux/1 -> BusCreator/1  "PTC GearBoxM_In0 GearNo"
  BusCreator/1 -> Out/1
  In/1 -> Demux/1

== system PTControl/CarMaker/IPG Vehicle/PowerTrain/PTControl Example/PTControl_In/CreateBus PTC GearBoxM_In1 ==
  In : Inport
  BusCreator : BusCreator  Inputs=20
  Demux : Demux  Outputs=20
  Out : Outport
  wires:
  Demux/20 -> BusCreator/20  "PTC GearBoxM_In1 Clutch_dis i_TrqIn2Out"
  Demux/19 -> BusCreator/19  "PTC GearBoxM_In1 Clutch_dis Trq_out"
  Demux/18 -> BusCreator/18  "PTC GearBoxM_In1 Clutch_dis Trq_in"
  Demux/17 -> BusCreator/17  "PTC GearBoxM_In1 Clutch_dis rotv_out"
  Demux/16 -> BusCreator/16  "PTC GearBoxM_In1 Clutch_dis rotv_in"
  Demux/15 -> BusCreator/15  "PTC GearBoxM_In1 Clutch_dis Pos"
  Demux/14 -> BusCreator/14  "PTC GearBoxM_In1 Clutch i_TrqIn2Out"
  Demux/13 -> BusCreator/13  "PTC GearBoxM_In1 Clutch Trq_out"
  Demux/12 -> BusCreator/12  "PTC GearBoxM_In1 Clutch Trq_in"
  Demux/11 -> BusCreator/11  "PTC GearBoxM_In1 Clutch rotv_out"
  Demux/10 -> BusCreator/10  "PTC GearBoxM_In1 Clutch rotv_in"
  Demux/9 -> BusCreator/9  "PTC GearBoxM_In1 Clutch Pos"
  Demux/8 -> BusCreator/8  "PTC GearBoxM_In1 Trq_out"
  Demux/7 -> BusCreator/7  "PTC GearBoxM_In1 Trq_in"
  Demux/6 -> BusCreator/6  "PTC GearBoxM_In1 rotv_out"
  Demux/5 -> BusCreator/5  "PTC GearBoxM_In1 rotv_in"
  Demux/4 -> BusCreator/4  "PTC GearBoxM_In1 i"
  Demux/3 -> BusCreator/3  "PTC GearBoxM_In1 Trq_DriveSrc_trg"
  Demux/2 -> BusCreator/2  "PTC GearBoxM_In1 GearNo_dis"
  Demux/1 -> BusCreator/1  "PTC GearBoxM_In1 GearNo"
  BusCreator/1 -> Out/1
  In/1 -> Demux/1

== system PTControl/CarMaker/IPG Vehicle/PowerTrain/PTControl Example/PTControl_In/CreateBus PTC GearBoxM_In2 ==
  In : Inport
  BusCreator : BusCreator  Inputs=20
  Demux : Demux  Outputs=20
  Out : Outport
  wires:
  Demux/20 -> BusCreator/20  "PTC GearBoxM_In2 Clutch_dis i_TrqIn2Out"
  Demux/19 -> BusCreator/19  "PTC GearBoxM_In2 Clutch_dis Trq_out"
  Demux/18 -> BusCreator/18  "PTC GearBoxM_In2 Clutch_dis Trq_in"
  Demux/17 -> BusCreator/17  "PTC GearBoxM_In2 Clutch_dis rotv_out"
  Demux/16 -> BusCreator/16  "PTC GearBoxM_In2 Clutch_dis rotv_in"
  Demux/15 -> BusCreator/15  "PTC GearBoxM_In2 Clutch_dis Pos"
  Demux/14 -> BusCreator/14  "PTC GearBoxM_In2 Clutch i_TrqIn2Out"
  Demux/13 -> BusCreator/13  "PTC GearBoxM_In2 Clutch Trq_out"
  Demux/12 -> BusCreator/12  "PTC GearBoxM_In2 Clutch Trq_in"
  Demux/11 -> BusCreator/11  "PTC GearBoxM_In2 Clutch rotv_out"
  Demux/10 -> BusCreator/10  "PTC GearBoxM_In2 Clutch rotv_in"
  Demux/9 -> BusCreator/9  "PTC GearBoxM_In2 Clutch Pos"
  Demux/8 -> BusCreator/8  "PTC GearBoxM_In2 Trq_out"
  Demux/7 -> BusCreator/7  "PTC GearBoxM_In2 Trq_in"
  Demux/6 -> BusCreator/6  "PTC GearBoxM_In2 rotv_out"
  Demux/5 -> BusCreator/5  "PTC GearBoxM_In2 rotv_in"
  Demux/4 -> BusCreator/4  "PTC GearBoxM_In2 i"
  Demux/3 -> BusCreator/3  "PTC GearBoxM_In2 Trq_DriveSrc_trg"
  Demux/2 -> BusCreator/2  "PTC GearBoxM_In2 GearNo_dis"
  Demux/1 -> BusCreator/1  "PTC GearBoxM_In2 GearNo"
  BusCreator/1 -> Out/1
  In/1 -> Demux/1

== system PTControl/CarMaker/IPG Vehicle/PowerTrain/PTControl Example/PTControl_In/CreateBus PTC GearBoxM_In3 ==
  In : Inport
  BusCreator : BusCreator  Inputs=20
  Demux : Demux  Outputs=20
  Out : Outport
  wires:
  Demux/20 -> BusCreator/20  "PTC GearBoxM_In3 Clutch_dis i_TrqIn2Out"
  Demux/19 -> BusCreator/19  "PTC GearBoxM_In3 Clutch_dis Trq_out"
  Demux/18 -> BusCreator/18  "PTC GearBoxM_In3 Clutch_dis Trq_in"
  Demux/17 -> BusCreator/17  "PTC GearBoxM_In3 Clutch_dis rotv_out"
  Demux/16 -> BusCreator/16  "PTC GearBoxM_In3 Clutch_dis rotv_in"
  Demux/15 -> BusCreator/15  "PTC GearBoxM_In3 Clutch_dis Pos"
  Demux/14 -> BusCreator/14  "PTC GearBoxM_In3 Clutch i_TrqIn2Out"
  Demux/13 -> BusCreator/13  "PTC GearBoxM_In3 Clutch Trq_out"
  Demux/12 -> BusCreator/12  "PTC GearBoxM_In3 Clutch Trq_in"
  Demux/11 -> BusCreator/11  "PTC GearBoxM_In3 Clutch rotv_out"
  Demux/10 -> BusCreator/10  "PTC GearBoxM_In3 Clutch rotv_in"
  Demux/9 -> BusCreator/9  "PTC GearBoxM_In3 Clutch Pos"
  Demux/8 -> BusCreator/8  "PTC GearBoxM_In3 Trq_out"
  Demux/7 -> BusCreator/7  "PTC GearBoxM_In3 Trq_in"
  Demux/6 -> BusCreator/6  "PTC GearBoxM_In3 rotv_out"
  Demux/5 -> BusCreator/5  "PTC GearBoxM_In3 rotv_in"
  Demux/4 -> BusCreator/4  "PTC GearBoxM_In3 i"
  Demux/3 -> BusCreator/3  "PTC GearBoxM_In3 Trq_DriveSrc_trg"
  Demux/2 -> BusCreator/2  "PTC GearBoxM_In3 GearNo_dis"
  Demux/1 -> BusCreator/1  "PTC GearBoxM_In3 GearNo"
  BusCreator/1 -> Out/1
  In/1 -> Demux/1

== system PTControl/CarMaker/IPG Vehicle/PowerTrain/PTControl Example/PTControl_In/CreateBus PTC ISGIn ==
  In : Inport
  BusCreator : BusCreator  Inputs=9
  Demux : Demux  Outputs=9
  Out : Outport
  wires:
  Demux/9 -> BusCreator/9  "PTC ISGIn i_M2W_RR"
  Demux/8 -> BusCreator/8  "PTC ISGIn i_M2W_RL"
  Demux/7 -> BusCreator/7  "PTC ISGIn i_M2W_FR"
  Demux/6 -> BusCreator/6  "PTC ISGIn i_M2W_FL"
  Demux/5 -> BusCreator/5  "PTC ISGIn PwrElec"
  Demux/4 -> BusCreator/4  "PTC ISGIn TrqGen_max"
  Demux/3 -> BusCreator/3  "PTC ISGIn TrqMot_max"
  Demux/2 -> BusCreator/2  "PTC ISGIn Trq"
  Demux/1 -> BusCreator/1  "PTC ISGIn rotv"
  BusCreator/1 -> Out/1
  In/1 -> Demux/1

== system PTControl/CarMaker/IPG Vehicle/PowerTrain/PTControl Example/PTControl_In/CreateBus PTC MotorIn0 ==
  In : Inport
  BusCreator : BusCreator  Inputs=9
  Demux : Demux  Outputs=9
  Out : Outport
  wires:
  Demux/9 -> BusCreator/9  "PTC MotorIn0 i_M2W_RR"
  Demux/8 -> BusCreator/8  "PTC MotorIn0 i_M2W_RL"
  Demux/7 -> BusCreator/7  "PTC MotorIn0 i_M2W_FR"
  Demux/6 -> BusCreator/6  "PTC MotorIn0 i_M2W_FL"
  Demux/5 -> BusCreator/5  "PTC MotorIn0 PwrElec"
  Demux/4 -> BusCreator/4  "PTC MotorIn0 TrqGen_max"
  Demux/3 -> BusCreator/3  "PTC MotorIn0 TrqMot_max"
  Demux/2 -> BusCreator/2  "PTC MotorIn0 Trq"
  Demux/1 -> BusCreator/1  "PTC MotorIn0 rotv"
  BusCreator/1 -> Out/1
  In/1 -> Demux/1

== system PTControl/CarMaker/IPG Vehicle/PowerTrain/PTControl Example/PTControl_In/CreateBus PTC MotorIn1 ==
  In : Inport
  BusCreator : BusCreator  Inputs=9
  Demux : Demux  Outputs=9
  Out : Outport
  wires:
  Demux/9 -> BusCreator/9  "PTC MotorIn1 i_M2W_RR"
  Demux/8 -> BusCreator/8  "PTC MotorIn1 i_M2W_RL"
  Demux/7 -> BusCreator/7  "PTC MotorIn1 i_M2W_FR"
  Demux/6 -> BusCreator/6  "PTC MotorIn1 i_M2W_FL"
  Demux/5 -> BusCreator/5  "PTC MotorIn1 PwrElec"
  Demux/4 -> BusCreator/4  "PTC MotorIn1 TrqGen_max"
  Demux/3 -> BusCreator/3  "PTC MotorIn1 TrqMot_max"
  Demux/2 -> BusCreator/2  "PTC MotorIn1 Trq"
  Demux/1 -> BusCreator/1  "PTC MotorIn1 rotv"
  BusCreator/1 -> Out/1
  In/1 -> Demux/1

== system PTControl/CarMaker/IPG Vehicle/PowerTrain/PTControl Example/PTControl_In/CreateBus PTC MotorIn2 ==
  In : Inport
  BusCreator : BusCreator  Inputs=9
  Demux : Demux  Outputs=9
  Out : Outport
  wires:
  Demux/9 -> BusCreator/9  "PTC MotorIn2 i_M2W_RR"
  Demux/8 -> BusCreator/8  "PTC MotorIn2 i_M2W_RL"
  Demux/7 -> BusCreator/7  "PTC MotorIn2 i_M2W_FR"
  Demux/6 -> BusCreator/6  "PTC MotorIn2 i_M2W_FL"
  Demux/5 -> BusCreator/5  "PTC MotorIn2 PwrElec"
  Demux/4 -> BusCreator/4  "PTC MotorIn2 TrqGen_max"
  Demux/3 -> BusCreator/3  "PTC MotorIn2 TrqMot_max"
  Demux/2 -> BusCreator/2  "PTC MotorIn2 Trq"
  Demux/1 -> BusCreator/1  "PTC MotorIn2 rotv"
  BusCreator/1 -> Out/1
  In/1 -> Demux/1

== system PTControl/CarMaker/IPG Vehicle/PowerTrain/PTControl Example/PTControl_In/CreateBus PTC MotorIn3 ==
  In : Inport
  BusCreator : BusCreator  Inputs=9
  Demux : Demux  Outputs=9
  Out : Outport
  wires:
  Demux/9 -> BusCreator/9  "PTC MotorIn3 i_M2W_RR"
  Demux/8 -> BusCreator/8  "PTC MotorIn3 i_M2W_RL"
  Demux/7 -> BusCreator/7  "PTC MotorIn3 i_M2W_FR"
  Demux/6 -> BusCreator/6  "PTC MotorIn3 i_M2W_FL"
  Demux/5 -> BusCreator/5  "PTC MotorIn3 PwrElec"
  Demux/4 -> BusCreator/4  "PTC MotorIn3 TrqGen_max"
  Demux/3 -> BusCreator/3  "PTC MotorIn3 TrqMot_max"
  Demux/2 -> BusCreator/2  "PTC MotorIn3 Trq"
  Demux/1 -> BusCreator/1  "PTC MotorIn3 rotv"
  BusCreator/1 -> Out/1
  In/1 -> Demux/1

== system PTControl/CarMaker/IPG Vehicle/PowerTrain/PTControl Example/PTControl_In/CreateBus PTC PwrSupplyIn ==
  In : Inport
  BusCreator : BusCreator  Inputs=12
  Demux : Demux  Outputs=12
  Out : Outport
  wires:
  Demux/12 -> BusCreator/12  "PTC PwrSupplyIn Eta_HV1toHV2"
  Demux/11 -> BusCreator/11  "PTC PwrSupplyIn Eta_HV1toLV"
  Demux/10 -> BusCreator/10  "PTC PwrSupplyIn Pwr_HV1toHV2_max"
  Demux/9 -> BusCreator/9  "PTC PwrSupplyIn Pwr_HV1toLV_max"
  Demux/8 -> BusCreator/8  "PTC PwrSupplyIn Pwr_HV1toHV2"
  Demux/7 -> BusCreator/7  "PTC PwrSupplyIn Pwr_HV1toLV"
  Demux/6 -> BusCreator/6  "PTC PwrSupplyIn Voltage_HV2"
  Demux/5 -> BusCreator/5  "PTC PwrSupplyIn Voltage_HV1"
  Demux/4 -> BusCreator/4  "PTC PwrSupplyIn Voltage_LV"
  Demux/3 -> BusCreator/3  "PTC PwrSupplyIn Pwr_HV2"
  Demux/2 -> BusCreator/2  "PTC PwrSupplyIn Pwr_HV1"
  Demux/1 -> BusCreator/1  "PTC PwrSupplyIn Pwr_LV"
  BusCreator/1 -> Out/1
  In/1 -> Demux/1
